simulink model "sys_sim"  (R2023a)
settings: Solver=FixedStepAuto  StartTime=0.0  StopTime=t_final  FixedStep=T  RelTol=1e-4
values from neighbouring files (symbols this model uses):
  A = A+0.2*c1*S_g*V_g    [params.m]
  B_u = [   zeros(4,2) ... (first row only)    [params.m]
  C = [1 0 -1  0 zeros(1,4) ... (first row only)    [params.m]
  n = size(A,1)    [params.m]
  noise_activation = 0    [params.m]
  S_g = S_eta    [params.m]
settings Model: Creator=20210012  LastModifiedBy=20210012
settings SolverCC: AlgebraicLoopSolver=TrustRegion
settings DataIOCC: SignalLogging=off  DSMLogging=off
settings DebuggingCC: UnconnectedInputMsg=warning  UnconnectedOutputMsg=warning  UnconnectedLineMsg=warning
settings ModelReferenceCC: EnableRefExpFcnMdlSchedulingChecks=on
settings SFSimCC: CustomCodeUndefinedFunction=UseInterfaceOnly
settings RTWCC: DLArmComputeVersion=19.05

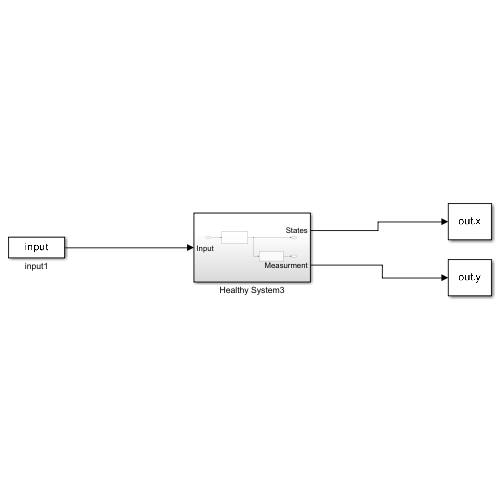
[thumbnail: Simulink's stored preview of the top-level diagram]
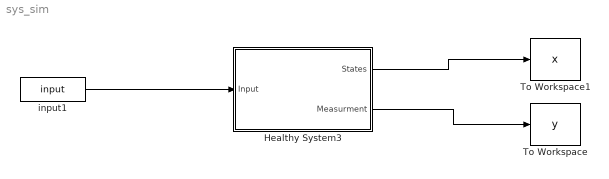
== system sys_sim ==
  Healthy System3 : Subsystem
  To Workspace : ToWorkspace  VariableName=y  SampleTime=-1
      settings: Save2DSignal=2-D array (concatenate along first dimension)
  To Workspace1 : ToWorkspace  VariableName=x  SampleTime=-1
      settings: Save2DSignal=2-D array (concatenate along first dimension)
  input1 : FromWorkspace  VariableName=input
  wires:
  Healthy System3/2(Measurment) -> To Workspace/1
  Healthy System3/1(States) -> To Workspace1/1
  input1/1 -> Healthy System3/1("Input ")

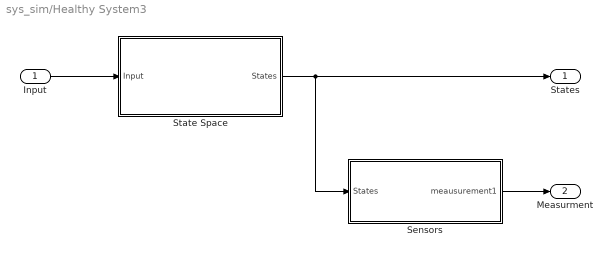
== system sys_sim/Healthy System3 ==
  "Input " : Inport
  Sensors : Subsystem
  State Space : Subsystem
  States : Outport  VectorParamsAs1DForOutWhenUnconnected=off
  Measurment : Outport  Port=2  VectorParamsAs1DForOutWhenUnconnected=off
  wires:
  State Space/1(States) -> States/1, Sensors/1(States)
  "Input "/1 -> State Space/1(" Input")
  Sensors/1(meausurement1) -> Measurment/1

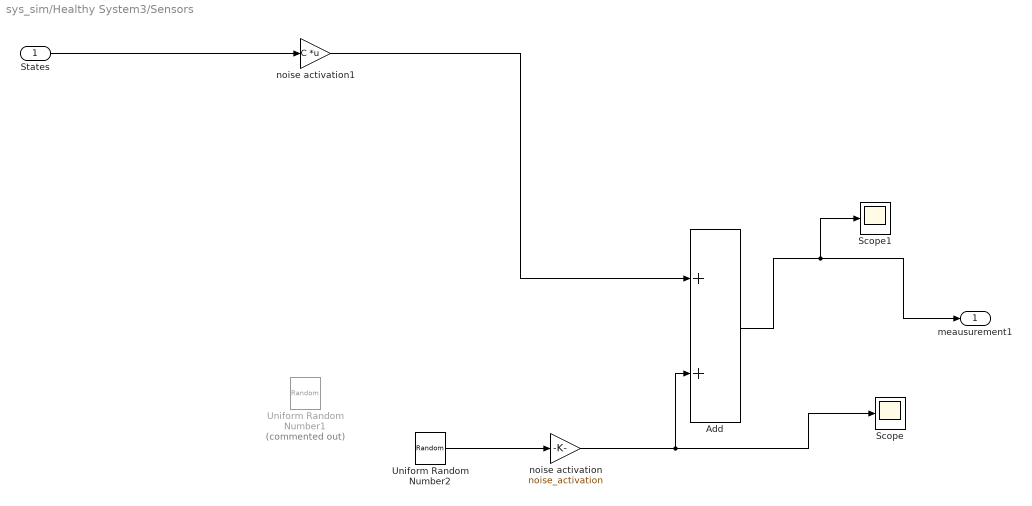
== system sys_sim/Healthy System3/Sensors ==
  States : Inport
  Add : Sum
  Scope : Scope
  Scope1 : Scope
  Uniform Random Number1 : UniformRandomNumber  Commented=on  Minimum=-[0.1; 0.1;0.1;0.1]*1e-3  Maximum=[0.1; 0.1;0.1;.1]*1e-3  SampleTime=1e-2
  Uniform Random Number2 : UniformRandomNumber  Minimum=-[0.005;0.005;0.04;0.04]/4  Maximum=[0.005;0.005;0.04;0.04]/4
  noise activation : Gain  Gain=noise_activation
  noise activation1 : Gain  Gain=C  Multiplication=Matrix(K*u)
  meausurement1 : Outport  VectorParamsAs1DForOutWhenUnconnected=off
  wires:
  States/1 -> noise activation1/1
  noise activation/1 -> Scope/1, Add/2
  noise activation1/1 -> Add/1
  Add/1 -> Scope1/1, meausurement1/1
  Uniform Random Number2/1 -> noise activation/1

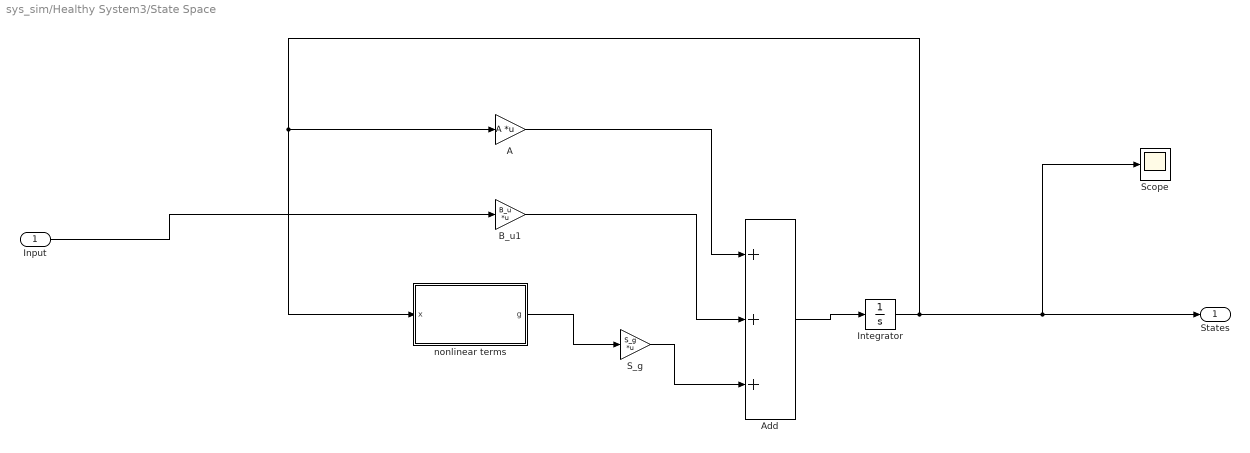
== system sys_sim/Healthy System3/State Space ==
  " Input" : Inport
  A : Gain  Gain=A  Multiplication=Matrix(K*u)
  Add : Sum  Inputs=+++
  B_u1 : Gain  Gain=B_u  Multiplication=Matrix(K*u)
  Integrator : Integrator  InitialCondition=1e-3*ones(n,1)
  S_g : Gain  Gain=S_g  Multiplication=Matrix(K*u)
  Scope : Scope
  "nonlinear terms " : MATLAB Function  TreatAsAtomicUnit=on
  States : Outport  VectorParamsAs1DForOutWhenUnconnected=off
  wires:
  Add/1 -> Integrator/1
  Integrator/1 -> "nonlinear terms "/1(x), A/1, Scope/1, States/1
  A/1 -> Add/1
  " Input"/1 -> B_u1/1
  B_u1/1 -> Add/2
  "nonlinear terms "/1(g) -> S_g/1
  S_g/1 -> Add/3

== matlab function sys_sim/Healthy System3/State Space/nonlinear terms  ==
  data: x input; g output
function g = g(x)

c1      = 710.70/1000*1e-3;
V_g   = [zeros(1,4) 10 0 -10  0
         zeros(1,4) 0 10  0 -10]; 

x_g = V_g*x;

g = c1*0.2*tanh(x_g);


end
